simulink model "v01_ssg_only"  (Simulink 7.5)
settings: Solver=ode45  StartTime=0.0  StopTime=128000  RelTol=1e-3
libraries: xbsIndex_r4 x439, xps_library x36, casper_library_misc x18, dspsigops x16, simulink x7
(part 1 of 5)
settings Model: Creator=mwagner  LastModifiedBy=gjones
settings DebuggingCC: StrictBusMsg=Warning

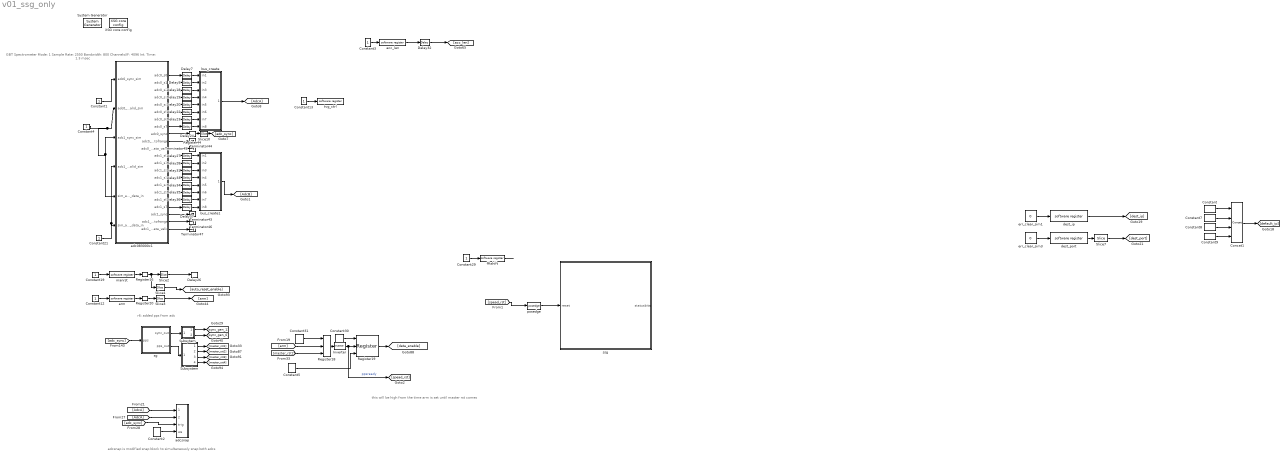
== system v01_ssg_only ==
  note: GBT Spectrometer
      | Mode: 1
      | Sample Rate: 2550
      | Bandwidth: 800
      | Channels/IF: 4096
      | Int. Time: 1.3 msec
  note: r6: added pps from adc
  note: adcsnap is modified snap block to simultaneously snap both adcs
  note: this will be high from the time arm is set until master rst comes
  " System Generator" : xbsIndex_r4/ System Generator  Tag=genX  SystemSampleTime=-1  xilinxfamily=virtex5  part=xc5vsx95t  speed=-1  package=ff1136  synthesis_tool=XST  clock_wrapper=Clock Enables  directory=./v01_ssg_only/sysgen  proj_type=Project Navigator  Synth_file=XST Defaults  Impl_file=ISE Defaults  testbench=off  simulink_period=1  sysclk_period=2.6667  dcm_input_clock_period=100  incr_netlist=off  trim_vbits=Everywhere in SubSystem  dbl_ovrd=According to Block Masks  core_generation=According to Block Masks  run_coregen=off  deprecated_control=off  eval_field=0  block_type=sysgen
      settings: block_version=10.1.3
  Concat1 : xbsIndex_r4/Concat  num_inputs=4  dbl_ovrd=off  block_type=concat
  Constant : xbsIndex_r4/Constant  const=10  gui_display_data_type=Fixed-point  arith_type=Unsigned  n_bits=8  bin_pt=0  preci_type=Single  exp_width=8  frac_width=24  explicit_period=on  period=1  equ=P=C  opselect=C  inp2=PCIN>>17  opr=+  inp1=P  carry=CIN  dbl_ovrd=off  block_type=constant
      settings: block_version=11.4
  Constant1 : Constant  SampleTime=1
  Constant{3,12..13,19,29} (5 alike) : Constant
  Constant{2,5,30..31} (4 alike) : xbsIndex_r4/Constant  const=1  gui_display_data_type=Fixed-point  arith_type=Boolean  n_bits=16  bin_pt=0  preci_type=Single  exp_width=8  frac_width=24  explicit_period=on  period=1  equ=P=C  opselect=C  inp2=PCIN>>17  opr=+  inp1=P  carry=CIN  dbl_ovrd=off  block_type=constant
      settings: block_version=11.4
  Constant21 : Constant  SampleTime=1
  Constant4 : Constant  SampleTime=1
  Constant7 : xbsIndex_r4/Constant  const=0  gui_display_data_type=Fixed-point  arith_type=Unsigned  n_bits=8  bin_pt=0  preci_type=Single  exp_width=8  frac_width=24  explicit_period=on  period=1  equ=P=C  opselect=C  inp2=PCIN>>17  opr=+  inp1=P  carry=CIN  dbl_ovrd=off  block_type=constant
      settings: block_version=11.4
  Constant8 : xbsIndex_r4/Constant  const=0  gui_display_data_type=Fixed-point  arith_type=Unsigned  n_bits=8  bin_pt=0  preci_type=Single  exp_width=8  frac_width=24  explicit_period=on  period=1  equ=P=C  opselect=C  inp2=PCIN>>17  opr=+  inp1=P  carry=CIN  dbl_ovrd=off  block_type=constant
      settings: block_version=11.4
  Constant9 : xbsIndex_r4/Constant  const=145  gui_display_data_type=Fixed-point  arith_type=Unsigned  n_bits=8  bin_pt=0  preci_type=Single  exp_width=8  frac_width=24  explicit_period=on  period=1  equ=P=C  opselect=C  inp2=PCIN>>17  opr=+  inp1=P  carry=CIN  dbl_ovrd=off  block_type=constant
      settings: block_version=11.4
  Delay{7,9,18..20,22..24,27..28,31,33..37} (16 alike) : xbsIndex_r4/Delay  rst=off  infoeditControl=Selection of Reset will increase slice count due to use of real FFs and instead of SRLs  en=off  latency=1  dbl_ovrd=off  reg_retiming=on  block_type=delay
      settings: block_version=11.4
  Delay26 : xbsIndex_r4/Delay  rst=off  infoeditControl=Selection of Reset will increase slice count due to use of real FFs and instead of SRLs  en=off  latency=8  dbl_ovrd=off  reg_retiming=on  block_type=delay
  Delay32 : xbsIndex_r4/Delay  rst=off  infoeditControl=Selection of Reset will increase slice count due to use of real FFs and instead of SRLs  en=off  latency=1  dbl_ovrd=off  reg_retiming=off  block_type=delay
      settings: block_version=11.4
  Inverter : xbsIndex_r4/Inverter  en=off  latency=0  dbl_ovrd=off  block_type=inv
      settings: block_version=11.4
  Register16 : xbsIndex_r4/Register  init=0  rst=off  en=off  dbl_ovrd=off  block_type=register
      settings: block_version=11.4
  Register18 : xbsIndex_r4/Register  init=0  rst=on  en=on  dbl_ovrd=off  block_type=register
      settings: block_version=11.4
  Register19 : xbsIndex_r4/Register  init=0  rst=on  en=on  dbl_ovrd=off  block_type=register
      settings: block_version=11.4
  Register20 : xbsIndex_r4/Register  init=0  rst=off  en=off  dbl_ovrd=off  block_type=register
      settings: block_version=11.4
  Register44 : xbsIndex_r4/Register  init=0  rst=off  en=off  dbl_ovrd=off  block_type=register
      settings: block_version=11.4
  Slice10 : xbsIndex_r4/Slice  nbits=1  boolean_output=on  mode=Lower Bit Location + Width  bit1=0  base1=MSB of Input  bit0=0  base0=LSB of Input  dbl_ovrd=off  block_type=slice
      settings: infoedit="Extracts a given range of bits from each input sample and presents it at the output.  The output type is ordinarily unsigned with binary point at zero, but can be Boolean when the slice is one bit wide.<P><P>Hardware notes: In hardware this block costs nothing."  block_version=10.1.3
  Slice2 : xbsIndex_r4/Slice  nbits=1  boolean_output=on  mode=Lower Bit Location + Width  bit1=0  base1=MSB of Input  bit0=0  base0=LSB of Input  dbl_ovrd=off  block_type=slice
      settings: block_version=10.1.3
  Slice3 : xbsIndex_r4/Slice  nbits=1  boolean_output=on  mode=Lower Bit Location + Width  bit1=0  base1=MSB of Input  bit0=0  base0=LSB of Input  dbl_ovrd=off  block_type=slice
      settings: block_version=10.1.3
  Slice4 : xbsIndex_r4/Slice  nbits=1  boolean_output=on  mode=Lower Bit Location + Width  bit1=0  base1=MSB of Input  bit0=1  base0=LSB of Input  dbl_ovrd=off  block_type=slice
      settings: block_version=10.1.3
  Slice7 : xbsIndex_r4/Slice  nbits=16  boolean_output=off  mode=Lower Bit Location + Width  bit1=0  base1=MSB of Input  bit0=0  base0=LSB of Input  dbl_ovrd=off  block_type=slice
      settings: infoedit="Extracts a given range of bits from each input sample and presents it at the output.  The output type is ordinarily unsigned with binary point at zero, but can be Boolean when the slice is one bit wide.<P><P>Hardware notes: In hardware this block costs nothing."  block_version=10.1.3
  Subsystem : Subsystem
  Subsytem : Subsystem
  Terminator{43..47} (5 alike) : Terminator
  XSG core config : xps_library/XSG core config  Tag=xps:xsg  SystemSampleTime=-1  hw_sys=ROACH:sx95t  ibob_linux=off  clk_src=adc0_clk  iBOB_clk_src=adc0_clk  BEE2_ctrl_clk_src=sys_clk  BEE2_usr_clk_src=sys_clk  ROACH_clk_src=adc0_clk  ROACH2_clk_src=adc0_clk  CORR_clk_src=sys_clk  gpio_clk_io_group=iBOB:sma  gpio_clk_bit_index=0  clk_rate=375  sample_period=1  synthesis_tool=XST  mpc_type=powerpc440_ext
  acc_len : xps_library/software register  Tag=xps:sw_reg  SystemSampleTime=-1  io_dir=From Processor  arith_type=Unsigned  bitwidth=32  bin_pt=0  sample_period=1  gw_name=v01_ssg_only_acc_len_user_data_out
      link override convert: arith_type=Unsigned  n_bits=32  bin_pt=0
      link override r_spec_2048_r102_cnt_rst_user_data_out: arith_type=Unsigned  n_bits=32  bin_pt=0  period=1
      link override r_spec_2048_r102_nosim_cnt_rst_user_data_out: arith_type=Unsigned  n_bits=32  bin_pt=0  period=1
      link override r_spec_2048_r103_cnt_rst_user_data_out: arith_type=Unsigned  n_bits=32  bin_pt=0  period=1
      link override roach_spec_no10gbe_sync_cnt_rst_user_data_out: arith_type=Unsigned  n_bits=32  bin_pt=0  period=1
      link override roach_spec_rst_cnt_user_data_out: arith_type=Unsigned  n_bits=32  bin_pt=0  period=1
      link override roach_spec_rst_sync_cnt_user_data_out: arith_type=Unsigned  n_bits=32  bin_pt=0  period=1
  adc083000x1 : Subsystem  Tag=xps:adc083000x2  AncestorBlock=xps_library/adc083000x2  mask(adc_083000x2){use_adc0=on, use_adc1=on, demux_adc=off, clock_sync=off, verbose=off, using_ctrl=on, adc_clk_rate=1500, sample_period=1, bit_width=8}
      mask prompts: use_adc0 "Use ZD0K0?"; use_adc1 "Use ZDOK1?"; demux_adc "Demux ADCs by 2?"; clock_sync "Interleave 2 ADC boards?"; verbose "Verbose Block Creation?"; using_ctrl "Add ports for control registers?"; adc_clk_rate "ADC clock rate (MHz)"; sample_period "Sample Period"; bit_width "Output Bit Width"
      mask help:
      | The ADC block converts analog inputs to digital outputs.
      | Every clock cycle, the inputs are sampled and digitized to
      | 8 bit binary point numbers in the range of [-1, 1).
      |
      | Online block-specific documentation: http://casper.berkeley.edu/wiki/Adc083000
      mask init:
      | adc083000_mask;
      mask Help: eval('xlWeb([getenv(''MLIB_ROOT''), ''\doc\html\sys_adc\sys_adc.html''])')
  adcsnap : Subsystem  mask(snap64){nsamples=11}
      mask prompts: nsamples "No. of samples(2^?)"
      mask help:
      | The <i>snap</i> block provides a packaged solution to capturing data from
      | the FPGA fabric and making it accessible from the CPU.  The block comes in
      | 2 flavors: <i>snap</i> (which captures to a 32 bit wide Shared BRAM), and
      | <i>snap64</i> (which captures to 2x32 bit wide Shared BRAMs to effect a
      | 64 bit capture).
      mask Help: eval('xlWeb(''http://casper.berkeley.edu/wiki/Snap'')')
  arm : xps_library/software register  Tag=xps:sw_reg  SystemSampleTime=-1  io_dir=From Processor  arith_type=Unsigned  bitwidth=32  bin_pt=0  sample_period=1  gw_name=v01_ssg_only_arm_user_data_out
      link override convert: arith_type=Unsigned  n_bits=32  bin_pt=0
      link override r_spec_2048_r102_cnt_rst_user_data_out: arith_type=Unsigned  n_bits=32  bin_pt=0  period=1
      link override r_spec_2048_r102_nosim_cnt_rst_user_data_out: arith_type=Unsigned  n_bits=32  bin_pt=0  period=1
      link override r_spec_2048_r103_cnt_rst_user_data_out: arith_type=Unsigned  n_bits=32  bin_pt=0  period=1
      link override roach_spec_no10gbe_sync_cnt_rst_user_data_out: arith_type=Unsigned  n_bits=32  bin_pt=0  period=1
      link override roach_spec_rst_cnt_user_data_out: arith_type=Unsigned  n_bits=32  bin_pt=0  period=1
      link override roach_spec_rst_sync_cnt_user_data_out: arith_type=Unsigned  n_bits=32  bin_pt=0  period=1
  bus_create : Subsystem  AncestorBlock=casper_library_flow_control/bus_create  mask(bus_create){inputNum=8}
      mask prompts: inputNum "Number of inputs:"
      mask init:
      | bus_create_init(gcb,...
      |     'inputNum', inputNum);
  bus_create1 : Subsystem  AncestorBlock=casper_library_flow_control/bus_create  mask(bus_create){inputNum=8}
      mask prompts: inputNum "Number of inputs:"
      mask init:
      | bus_create_init(gcb,...
      |     'inputNum', inputNum);
  dest_ip : xps_library/software register  Tag=xps:sw_reg  SystemSampleTime=-1  io_dir=From Processor  arith_type=Unsigned  bitwidth=32  bin_pt=0  sample_period=1  gw_name=v01_ssg_only_dest_ip_user_data_out
      link override r_10gbe_demo_dest_ip_user_data_out: arith_type=Unsigned  n_bits=32  bin_pt=0  period=1
      link override r_10gbe_test_dest_ip_user_data_out: arith_type=Unsigned  n_bits=32  bin_pt=0  period=1
      link override r_xaui_test_cnt_rst_user_data_out: arith_type=Unsigned  n_bits=32  bin_pt=0  period=1
  dest_port : xps_library/software register  Tag=xps:sw_reg  SystemSampleTime=-1  io_dir=From Processor  arith_type=Unsigned  bitwidth=32  bin_pt=0  sample_period=1  gw_name=v01_ssg_only_dest_port_user_data_out
      link override r_10gbe_demo_dest_port_user_data_out: arith_type=Unsigned  n_bits=32  bin_pt=0  period=1
      link override r_10gbe_test_dest_port_user_data_out: arith_type=Unsigned  n_bits=32  bin_pt=0  period=1
      link override r_xaui_test_cnt_rst_user_data_out: arith_type=Unsigned  n_bits=32  bin_pt=0  period=1
  err_clear_sim1 : Constant  Value=0
  err_clear_sim3 : Constant  Value=0
  fftshift : xps_library/software register  Tag=xps:sw_reg  SystemSampleTime=-1  io_dir=From Processor  arith_type=Unsigned  bitwidth=32  bin_pt=0  sample_period=1  gw_name=v01_ssg_only_fftshift_user_data_out
  manrst : xps_library/software register  Tag=xps:sw_reg  SystemSampleTime=-1  io_dir=From Processor  arith_type=Unsigned  bitwidth=32  bin_pt=0  sample_period=1  gw_name=v01_ssg_only_manrst_user_data_out
      link override convert: arith_type=Unsigned  n_bits=32  bin_pt=0
      link override r_spec_2048_r102_cnt_rst_user_data_out: arith_type=Unsigned  n_bits=32  bin_pt=0  period=1
      link override r_spec_2048_r102_nosim_cnt_rst_user_data_out: arith_type=Unsigned  n_bits=32  bin_pt=0  period=1
      link override r_spec_2048_r103_cnt_rst_user_data_out: arith_type=Unsigned  n_bits=32  bin_pt=0  period=1
      link override roach_spec_no10gbe_sync_cnt_rst_user_data_out: arith_type=Unsigned  n_bits=32  bin_pt=0  period=1
      link override roach_spec_rst_cnt_user_data_out: arith_type=Unsigned  n_bits=32  bin_pt=0  period=1
      link override roach_spec_rst_sync_cnt_user_data_out: arith_type=Unsigned  n_bits=32  bin_pt=0  period=1
  posedge : casper_library_misc/posedge  Tag=Rising Edge Detector  SystemSampleTime=-1
  sg : Subsystem
  ssg : Subsystem
  tvg_ctrl : xps_library/software register  Tag=xps:sw_reg  SystemSampleTime=-1  io_dir=From Processor  arith_type=Unsigned  bitwidth=32  bin_pt=0  sample_period=1  gw_name=v01_ssg_only_tvg_ctrl_user_data_out
      link override convert: arith_type=Unsigned  n_bits=32  bin_pt=0
      link override r_spec_2048_r102_cnt_rst_user_data_out: arith_type=Unsigned  n_bits=32  bin_pt=0  period=1
      link override r_spec_2048_r102_nosim_cnt_rst_user_data_out: arith_type=Unsigned  n_bits=32  bin_pt=0  period=1
      link override r_spec_2048_r103_cnt_rst_user_data_out: arith_type=Unsigned  n_bits=32  bin_pt=0  period=1
      link override roach_spec_no10gbe_sync_cnt_rst_user_data_out: arith_type=Unsigned  n_bits=32  bin_pt=0  period=1
      link override roach_spec_rst_cnt_user_data_out: arith_type=Unsigned  n_bits=32  bin_pt=0  period=1
      link override roach_spec_rst_sync_cnt_user_data_out: arith_type=Unsigned  n_bits=32  bin_pt=0  period=1
  wires:
  manrst/1 -> Register16/1
  Constant19/1 -> manrst/1
  Register16/1 -> Slice2/1, Slice4/1
  Slice2/1 -> Delay26/1
  Constant4/1 -> adc083000x1/2(adc0_data_valid_sim), adc083000x1/3(adc1_sync_sim), adc083000x1/5(sim_adc0_data_in)
  Constant1/1 -> adc083000x1/1(adc0_sync_sim)
  Slice10/1 -> [adc_sync]
  Register44/1 -> Slice10/1
  Constant21/1 -> adc083000x1/4(adc1_data_valid_sim), adc083000x1/6(sim_adc1_data_in)
  Concat1/1 -> [default_ip]
  acc_len/1 -> Delay32/1
  Constant3/1 -> acc_len/1
  Delay32/1 -> [acc_len]
  err_clear_sim1/1 -> dest_ip/1
  dest_ip/1 -> [dest_ip]
  dest_port/1 -> Slice7/1
  err_clear_sim3/1 -> dest_port/1
  Slice7/1 -> [dest_port]
  Constant/1 -> Concat1/1
  Constant7/1 -> Concat1/2
  Constant8/1 -> Concat1/3
  Constant9/1 -> Concat1/4
  Constant30/1 -> Register19/1
  Register18/1 -> Inverter/1
  Inverter/1 -> Register19/2, [spead_rst]  "ppsready"
  Constant31/1 -> Register18/1
  arm/1 -> Register20/1
  Constant12/1 -> arm/1
  Register20/1 -> Slice3/1
  Slice3/1 -> [arm]
  [arm] -> Register18/2
  [master_rst2] -> Register18/3
  Constant5/1 -> Register19/3
  Register19/1 -> [data_enable]
  [adc_sync] -> sg/1(pps)
  Slice4/1 -> [auto_reset_enable]
  sg/1(sync_out) -> Subsytem/1(In1)
  Subsytem/1(Out1) -> [sync_gen_1]
  Subsytem/2(Out2) -> [sync_gen_0]
  Delay7/1 -> bus_create/1(in1)
  Delay9/1 -> bus_create/2(in2)
  Delay18/1 -> bus_create/3(in3)
  Delay19/1 -> bus_create/4(in4)
  Delay20/1 -> bus_create/5(in5)
  Delay22/1 -> bus_create/6(in6)
  Delay23/1 -> bus_create/7(in7)
  Delay24/1 -> bus_create/8(in8)
  Delay27/1 -> bus_create1/1(in1)
  Delay28/1 -> bus_create1/2(in2)
  Delay31/1 -> bus_create1/3(in3)
  Delay33/1 -> bus_create1/4(in4)
  Delay34/1 -> bus_create1/5(in5)
  Delay35/1 -> bus_create1/6(in6)
  Delay36/1 -> bus_create1/7(in7)
  Delay37/1 -> bus_create1/8(in8)
  sg/2(pps_out) -> Subsystem/1(In2)
  Subsystem/1(Out1) -> [master_rst1]
  Subsystem/2(Out2) -> [master_rst2]
  Subsystem/3(Out3) -> [master_rst3]
  Subsystem/4(Out4) -> [master_rst4]
  adc083000x1/1(adc0_s0) -> Delay7/1
  adc083000x1/2(adc0_s1) -> Delay9/1
  adc083000x1/3(adc0_s2) -> Delay18/1
  adc083000x1/4(adc0_s3) -> Delay19/1
  adc083000x1/5(adc0_s4) -> Delay20/1
  adc083000x1/6(adc0_s5) -> Delay22/1
  adc083000x1/7(adc0_s6) -> Delay23/1
  adc083000x1/8(adc0_s7) -> Delay24/1
  adc083000x1/9(adc0_sync) -> Register44/1
  adc083000x1/10(adc0_outofrange) -> Terminator44/1
  adc083000x1/11(adc0_data_valid) -> Terminator45/1
  adc083000x1/12(adc1_s0) -> Delay27/1
  adc083000x1/13(adc1_s1) -> Delay28/1
  adc083000x1/14(adc1_s2) -> Delay31/1
  adc083000x1/15(adc1_s3) -> Delay33/1
  adc083000x1/16(adc1_s4) -> Delay34/1
  adc083000x1/17(adc1_s5) -> Delay35/1
  adc083000x1/18(adc1_s6) -> Delay36/1
  adc083000x1/19(adc1_s7) -> Delay37/1
  adc083000x1/20(adc1_sync) -> Terminator43/1
  adc083000x1/21(adc1_outofrange) -> Terminator46/1
  adc083000x1/22(adc1_data_valid) -> Terminator47/1
  Constant13/1 -> tvg_ctrl/1
  bus_create/1(bus_out) -> [AdcA]
  bus_create1/1(bus_out) -> [AdcB]
  Constant29/1 -> fftshift/1
  fftshift/1 -> ?
  [AdcA] -> adcsnap/1(adcA)
  [AdcA] -> adcsnap/2(adcB)
  [adc_sync] -> adcsnap/3(trig)
  Constant2/1 -> adcsnap/4(we)
  ? -> ?
  ? -> ?
  ? -> ?
  [spead_rst] -> posedge/1
  posedge/1 -> ssg/1(reset)

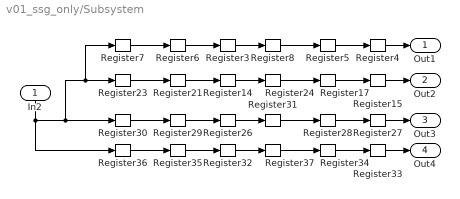
== system v01_ssg_only/Subsystem ==
  In2 : Inport
  Register{3..8,14..15,17,21,23..24,26..37} (24 alike) : xbsIndex_r4/Register  init=0  rst=off  en=off  dbl_ovrd=off  block_type=register
      settings: block_version=11.4
  Out1 : Outport
  Out2 : Outport  Port=2
  Out3 : Outport  Port=3
  Out4 : Outport  Port=4
  wires:
  Register7/1 -> Register6/1
  Register6/1 -> Register3/1
  Register8/1 -> Register5/1
  Register5/1 -> Register4/1
  Register3/1 -> Register8/1
  Register23/1 -> Register21/1
  Register21/1 -> Register14/1
  Register24/1 -> Register17/1
  Register17/1 -> Register15/1
  Register14/1 -> Register24/1
  Register30/1 -> Register29/1
  Register29/1 -> Register26/1
  Register31/1 -> Register28/1
  Register28/1 -> Register27/1
  Register26/1 -> Register31/1
  Register36/1 -> Register35/1
  Register35/1 -> Register32/1
  Register37/1 -> Register34/1
  Register34/1 -> Register33/1
  Register32/1 -> Register37/1
  In2/1 -> Register36/1, Register30/1, Register23/1, Register7/1
  Register4/1 -> Out1/1
  Register15/1 -> Out2/1
  Register27/1 -> Out3/1
  Register33/1 -> Out4/1

== system v01_ssg_only/Subsytem ==
  In1 : Inport
  Register{3..8,14..15,17} (9 alike) : xbsIndex_r4/Register  init=0  rst=off  en=off  dbl_ovrd=off  block_type=register
      settings: block_version=11.4
  Out1 : Outport
  Out2 : Outport  Port=2
  wires:
  Register3/1 -> Register4/1, Register5/1
  Register7/1 -> Register6/1
  Register6/1 -> Register3/1
  Register5/1 -> Register14/1
  Register4/1 -> Register8/1
  Register8/1 -> Register17/1
  Register14/1 -> Register15/1
  Register17/1 -> Out1/1
  In1/1 -> Register7/1
  Register15/1 -> Out2/1

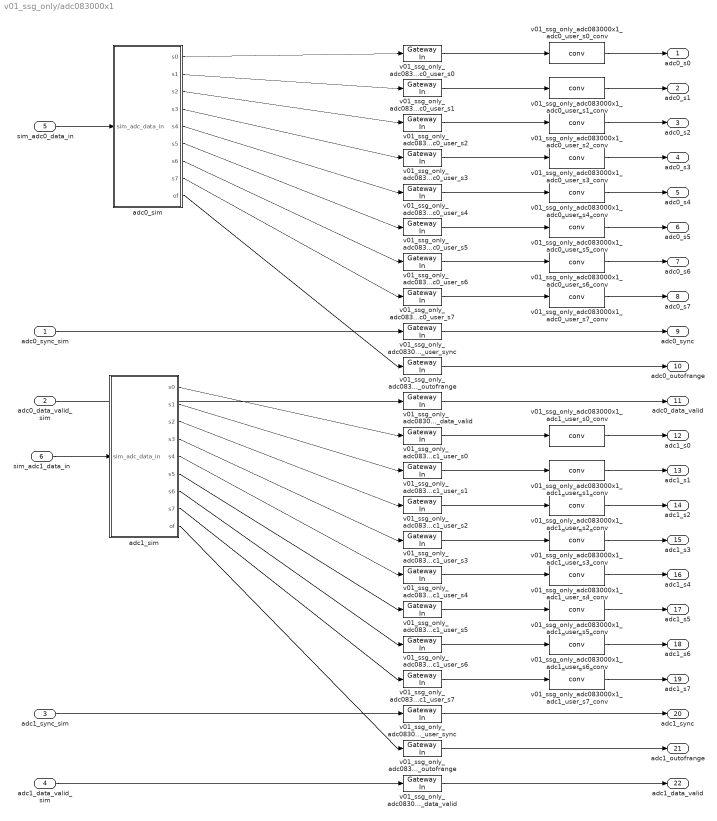
== system v01_ssg_only/adc083000x1 ==
  adc0_sync_sim : Inport
  adc0_data_valid_sim : Inport  Port=2
  adc1_sync_sim : Inport  Port=3
  adc1_data_valid_sim : Inport  Port=4
  sim_adc0_data_in : Inport  Port=5
  sim_adc1_data_in : Inport  Port=6
  adc0_sim : Subsystem  AncestorBlock=xps_library/ADCs/adc_sim  mask(adc_sim){nStreams=8, bit_width=8}
      mask prompts: nStreams "Number of Output Streams"; bit_width "Sample Bit Width"
      mask help:
      | This block simulates the behavior of a demuxed ADC, which takes
      | as input a waveform and returns digital samples in parallel at
      | a slower rate.
      |
      | This block is used to simulate the behavior
      mask init:
      | adc_sim_init(gcb, ...
      |     'nStreams', nStreams, ...
      |     'bit_width', bit_width);
  adc1_sim : Subsystem  AncestorBlock=xps_library/ADCs/adc_sim  mask(adc_sim){nStreams=8, bit_width=8}
      mask prompts: nStreams "Number of Output Streams"; bit_width "Sample Bit Width"
      mask help:
      | This block simulates the behavior of a demuxed ADC, which takes
      | as input a waveform and returns digital samples in parallel at
      | a slower rate.
      |
      | This block is used to simulate the behavior
      mask init:
      | adc_sim_init(gcb, ...
      |     'nStreams', nStreams, ...
      |     'bit_width', bit_width);
  v01_ssg_only_adc083000x1_adc0_user_data_valid : xbsIndex_r4/Gateway In  gui_display_data_type=Fixed-point  arith_type=Unsigned  n_bits=1  bin_pt=0  preci_type=Single  exp_width=8  frac_width=24  quantization="Round  (unbiased: +/- Inf)"  overflow=Saturate  period=1  dbl_ovrd=off  timing_constraint=None  locs_specified=off  LOCs={}  hdl_port=on  block_type=gatewayin
      settings: infoedit="Gateway in block.  Converts inputs of type Simulink integer, double and fixed point to  Xilinx fixed point or floating-point data type.<br><br>Hardware notes:  In hardware these blocks become top level input ports."
  v01_ssg_only_adc083000x1_adc0_user_outofrange : xbsIndex_r4/Gateway In  gui_display_data_type=Fixed-point  arith_type=Unsigned  n_bits=4  bin_pt=0  preci_type=Single  exp_width=8  frac_width=24  quantization="Round  (unbiased: +/- Inf)"  overflow=Saturate  period=1  dbl_ovrd=off  timing_constraint=None  locs_specified=off  LOCs={}  hdl_port=on  block_type=gatewayin
      settings: infoedit="Gateway in block.  Converts inputs of type Simulink integer, double and fixed point to  Xilinx fixed point or floating-point data type.<br><br>Hardware notes:  In hardware these blocks become top level input ports."
  v01_ssg_only_adc083000x1_adc0_user_s{0..7} (8 alike) : xbsIndex_r4/Gateway In  gui_display_data_type=Fixed-point  arith_type=Unsigned  n_bits=8  bin_pt=0  preci_type=Single  exp_width=8  frac_width=24  quantization="Round  (unbiased: +/- Inf)"  overflow=Saturate  period=1  dbl_ovrd=off  timing_constraint=None  locs_specified=off  LOCs={}  hdl_port=on  block_type=gatewayin
      settings: infoedit="Gateway in block.  Converts inputs of type Simulink integer, double and fixed point to  Xilinx fixed point or floating-point data type.<br><br>Hardware notes:  In hardware these blocks become top level input ports."
  v01_ssg_only_adc083000x1_adc0_user_s0_conv : xps_library/ADCs/conv  SystemSampleTime=-1  bit_width=8
  v01_ssg_only_adc083000x1_adc0_user_s1_conv : xps_library/ADCs/conv  SystemSampleTime=-1  bit_width=8
  v01_ssg_only_adc083000x1_adc0_user_s2_conv : xps_library/ADCs/conv  SystemSampleTime=-1  bit_width=8
  v01_ssg_only_adc083000x1_adc0_user_s3_conv : xps_library/ADCs/conv  SystemSampleTime=-1  bit_width=8
  v01_ssg_only_adc083000x1_adc0_user_s4_conv : xps_library/ADCs/conv  SystemSampleTime=-1  bit_width=8
  v01_ssg_only_adc083000x1_adc0_user_s5_conv : xps_library/ADCs/conv  SystemSampleTime=-1  bit_width=8
  v01_ssg_only_adc083000x1_adc0_user_s6_conv : xps_library/ADCs/conv  SystemSampleTime=-1  bit_width=8
  v01_ssg_only_adc083000x1_adc0_user_s7_conv : xps_library/ADCs/conv  SystemSampleTime=-1  bit_width=8
  v01_ssg_only_adc083000x1_adc0_user_sync : xbsIndex_r4/Gateway In  gui_display_data_type=Fixed-point  arith_type=Unsigned  n_bits=4  bin_pt=0  preci_type=Single  exp_width=8  frac_width=24  quantization="Round  (unbiased: +/- Inf)"  overflow=Saturate  period=1  dbl_ovrd=off  timing_constraint=None  locs_specified=off  LOCs={}  hdl_port=on  block_type=gatewayin
      settings: infoedit="Gateway in block.  Converts inputs of type Simulink integer, double and fixed point to  Xilinx fixed point or floating-point data type.<br><br>Hardware notes:  In hardware these blocks become top level input ports."
  v01_ssg_only_adc083000x1_adc1_user_data_valid : xbsIndex_r4/Gateway In  gui_display_data_type=Fixed-point  arith_type=Unsigned  n_bits=1  bin_pt=0  preci_type=Single  exp_width=8  frac_width=24  quantization="Round  (unbiased: +/- Inf)"  overflow=Saturate  period=1  dbl_ovrd=off  timing_constraint=None  locs_specified=off  LOCs={}  hdl_port=on  block_type=gatewayin
      settings: infoedit="Gateway in block.  Converts inputs of type Simulink integer, double and fixed point to  Xilinx fixed point or floating-point data type.<br><br>Hardware notes:  In hardware these blocks become top level input ports."
  v01_ssg_only_adc083000x1_adc1_user_outofrange : xbsIndex_r4/Gateway In  gui_display_data_type=Fixed-point  arith_type=Unsigned  n_bits=4  bin_pt=0  preci_type=Single  exp_width=8  frac_width=24  quantization="Round  (unbiased: +/- Inf)"  overflow=Saturate  period=1  dbl_ovrd=off  timing_constraint=None  locs_specified=off  LOCs={}  hdl_port=on  block_type=gatewayin
      settings: infoedit="Gateway in block.  Converts inputs of type Simulink integer, double and fixed point to  Xilinx fixed point or floating-point data type.<br><br>Hardware notes:  In hardware these blocks become top level input ports."
  v01_ssg_only_adc083000x1_adc1_user_s{0..7} (8 alike) : xbsIndex_r4/Gateway In  gui_display_data_type=Fixed-point  arith_type=Unsigned  n_bits=8  bin_pt=0  preci_type=Single  exp_width=8  frac_width=24  quantization="Round  (unbiased: +/- Inf)"  overflow=Saturate  period=1  dbl_ovrd=off  timing_constraint=None  locs_specified=off  LOCs={}  hdl_port=on  block_type=gatewayin
      settings: infoedit="Gateway in block.  Converts inputs of type Simulink integer, double and fixed point to  Xilinx fixed point or floating-point data type.<br><br>Hardware notes:  In hardware these blocks become top level input ports."
  v01_ssg_only_adc083000x1_adc1_user_s0_conv : xps_library/ADCs/conv  SystemSampleTime=-1  bit_width=8
  v01_ssg_only_adc083000x1_adc1_user_s1_conv : xps_library/ADCs/conv  SystemSampleTime=-1  bit_width=8
  v01_ssg_only_adc083000x1_adc1_user_s2_conv : xps_library/ADCs/conv  SystemSampleTime=-1  bit_width=8
  v01_ssg_only_adc083000x1_adc1_user_s3_conv : xps_library/ADCs/conv  SystemSampleTime=-1  bit_width=8
  v01_ssg_only_adc083000x1_adc1_user_s4_conv : xps_library/ADCs/conv  SystemSampleTime=-1  bit_width=8
  v01_ssg_only_adc083000x1_adc1_user_s5_conv : xps_library/ADCs/conv  SystemSampleTime=-1  bit_width=8
  v01_ssg_only_adc083000x1_adc1_user_s6_conv : xps_library/ADCs/conv  SystemSampleTime=-1  bit_width=8
  v01_ssg_only_adc083000x1_adc1_user_s7_conv : xps_library/ADCs/conv  SystemSampleTime=-1  bit_width=8
  v01_ssg_only_adc083000x1_adc1_user_sync : xbsIndex_r4/Gateway In  gui_display_data_type=Fixed-point  arith_type=Unsigned  n_bits=4  bin_pt=0  preci_type=Single  exp_width=8  frac_width=24  quantization="Round  (unbiased: +/- Inf)"  overflow=Saturate  period=1  dbl_ovrd=off  timing_constraint=None  locs_specified=off  LOCs={}  hdl_port=on  block_type=gatewayin
      settings: infoedit="Gateway in block.  Converts inputs of type Simulink integer, double and fixed point to  Xilinx fixed point or floating-point data type.<br><br>Hardware notes:  In hardware these blocks become top level input ports."
  adc0_s0 : Outport
  adc0_s1 : Outport  Port=2
  adc0_s2 : Outport  Port=3
  adc0_s3 : Outport  Port=4
  adc0_s4 : Outport  Port=5
  adc0_s5 : Outport  Port=6
  adc0_s6 : Outport  Port=7
  adc0_s7 : Outport  Port=8
  adc0_sync : Outport  Port=9
  adc0_outofrange : Outport  Port=10
  adc0_data_valid : Outport  Port=11
  adc1_s0 : Outport  Port=12
  adc1_s1 : Outport  Port=13
  adc1_s2 : Outport  Port=14
  adc1_s3 : Outport  Port=15
  adc1_s4 : Outport  Port=16
  adc1_s5 : Outport  Port=17
  adc1_s6 : Outport  Port=18
  adc1_s7 : Outport  Port=19
  adc1_sync : Outport  Port=20
  adc1_outofrange : Outport  Port=21
  adc1_data_valid : Outport  Port=22
  wires:
  sim_adc0_data_in/1 -> adc0_sim/1(sim_adc_data_in)
  sim_adc1_data_in/1 -> adc1_sim/1(sim_adc_data_in)
  adc0_sim/1(s0) -> v01_ssg_only_adc083000x1_adc0_user_s0/1
  v01_ssg_only_adc083000x1_adc0_user_s0/1 -> v01_ssg_only_adc083000x1_adc0_user_s0_conv/1
  v01_ssg_only_adc083000x1_adc0_user_s0_conv/1 -> adc0_s0/1
  adc0_sim/2(s1) -> v01_ssg_only_adc083000x1_adc0_user_s1/1
  v01_ssg_only_adc083000x1_adc0_user_s1/1 -> v01_ssg_only_adc083000x1_adc0_user_s1_conv/1
  v01_ssg_only_adc083000x1_adc0_user_s1_conv/1 -> adc0_s1/1
  adc0_sim/3(s2) -> v01_ssg_only_adc083000x1_adc0_user_s2/1
  v01_ssg_only_adc083000x1_adc0_user_s2/1 -> v01_ssg_only_adc083000x1_adc0_user_s2_conv/1
  v01_ssg_only_adc083000x1_adc0_user_s2_conv/1 -> adc0_s2/1
  adc0_sim/4(s3) -> v01_ssg_only_adc083000x1_adc0_user_s3/1
  v01_ssg_only_adc083000x1_adc0_user_s3/1 -> v01_ssg_only_adc083000x1_adc0_user_s3_conv/1
  v01_ssg_only_adc083000x1_adc0_user_s3_conv/1 -> adc0_s3/1
  adc0_sim/5(s4) -> v01_ssg_only_adc083000x1_adc0_user_s4/1
  v01_ssg_only_adc083000x1_adc0_user_s4/1 -> v01_ssg_only_adc083000x1_adc0_user_s4_conv/1
  v01_ssg_only_adc083000x1_adc0_user_s4_conv/1 -> adc0_s4/1
  adc0_sim/6(s5) -> v01_ssg_only_adc083000x1_adc0_user_s5/1
  v01_ssg_only_adc083000x1_adc0_user_s5/1 -> v01_ssg_only_adc083000x1_adc0_user_s5_conv/1
  v01_ssg_only_adc083000x1_adc0_user_s5_conv/1 -> adc0_s5/1
  adc0_sim/7(s6) -> v01_ssg_only_adc083000x1_adc0_user_s6/1
  v01_ssg_only_adc083000x1_adc0_user_s6/1 -> v01_ssg_only_adc083000x1_adc0_user_s6_conv/1
  v01_ssg_only_adc083000x1_adc0_user_s6_conv/1 -> adc0_s6/1
  adc0_sim/8(s7) -> v01_ssg_only_adc083000x1_adc0_user_s7/1
  v01_ssg_only_adc083000x1_adc0_user_s7/1 -> v01_ssg_only_adc083000x1_adc0_user_s7_conv/1
  v01_ssg_only_adc083000x1_adc0_user_s7_conv/1 -> adc0_s7/1
  adc0_sync_sim/1 -> v01_ssg_only_adc083000x1_adc0_user_sync/1
  v01_ssg_only_adc083000x1_adc0_user_sync/1 -> adc0_sync/1
  adc0_sim/9(of) -> v01_ssg_only_adc083000x1_adc0_user_outofrange/1
  v01_ssg_only_adc083000x1_adc0_user_outofrange/1 -> adc0_outofrange/1
  adc0_data_valid_sim/1 -> v01_ssg_only_adc083000x1_adc0_user_data_valid/1
  v01_ssg_only_adc083000x1_adc0_user_data_valid/1 -> adc0_data_valid/1
  adc1_sim/1(s0) -> v01_ssg_only_adc083000x1_adc1_user_s0/1
  v01_ssg_only_adc083000x1_adc1_user_s0/1 -> v01_ssg_only_adc083000x1_adc1_user_s0_conv/1
  v01_ssg_only_adc083000x1_adc1_user_s0_conv/1 -> adc1_s0/1
  adc1_sim/2(s1) -> v01_ssg_only_adc083000x1_adc1_user_s1/1
  v01_ssg_only_adc083000x1_adc1_user_s1/1 -> v01_ssg_only_adc083000x1_adc1_user_s1_conv/1
  v01_ssg_only_adc083000x1_adc1_user_s1_conv/1 -> adc1_s1/1
  adc1_sim/3(s2) -> v01_ssg_only_adc083000x1_adc1_user_s2/1
  v01_ssg_only_adc083000x1_adc1_user_s2/1 -> v01_ssg_only_adc083000x1_adc1_user_s2_conv/1
  v01_ssg_only_adc083000x1_adc1_user_s2_conv/1 -> adc1_s2/1
  adc1_sim/4(s3) -> v01_ssg_only_adc083000x1_adc1_user_s3/1
  v01_ssg_only_adc083000x1_adc1_user_s3/1 -> v01_ssg_only_adc083000x1_adc1_user_s3_conv/1
  v01_ssg_only_adc083000x1_adc1_user_s3_conv/1 -> adc1_s3/1
  adc1_sim/5(s4) -> v01_ssg_only_adc083000x1_adc1_user_s4/1
  v01_ssg_only_adc083000x1_adc1_user_s4/1 -> v01_ssg_only_adc083000x1_adc1_user_s4_conv/1
  v01_ssg_only_adc083000x1_adc1_user_s4_conv/1 -> adc1_s4/1
  adc1_sim/6(s5) -> v01_ssg_only_adc083000x1_adc1_user_s5/1
  v01_ssg_only_adc083000x1_adc1_user_s5/1 -> v01_ssg_only_adc083000x1_adc1_user_s5_conv/1
  v01_ssg_only_adc083000x1_adc1_user_s5_conv/1 -> adc1_s5/1
  adc1_sim/7(s6) -> v01_ssg_only_adc083000x1_adc1_user_s6/1
  v01_ssg_only_adc083000x1_adc1_user_s6/1 -> v01_ssg_only_adc083000x1_adc1_user_s6_conv/1
  v01_ssg_only_adc083000x1_adc1_user_s6_conv/1 -> adc1_s6/1
  adc1_sim/8(s7) -> v01_ssg_only_adc083000x1_adc1_user_s7/1
  v01_ssg_only_adc083000x1_adc1_user_s7/1 -> v01_ssg_only_adc083000x1_adc1_user_s7_conv/1
  v01_ssg_only_adc083000x1_adc1_user_s7_conv/1 -> adc1_s7/1
  adc1_sync_sim/1 -> v01_ssg_only_adc083000x1_adc1_user_sync/1
  v01_ssg_only_adc083000x1_adc1_user_sync/1 -> adc1_sync/1
  adc1_sim/9(of) -> v01_ssg_only_adc083000x1_adc1_user_outofrange/1
  v01_ssg_only_adc083000x1_adc1_user_outofrange/1 -> adc1_outofrange/1
  adc1_data_valid_sim/1 -> v01_ssg_only_adc083000x1_adc1_user_data_valid/1
  v01_ssg_only_adc083000x1_adc1_user_data_valid/1 -> adc1_data_valid/1

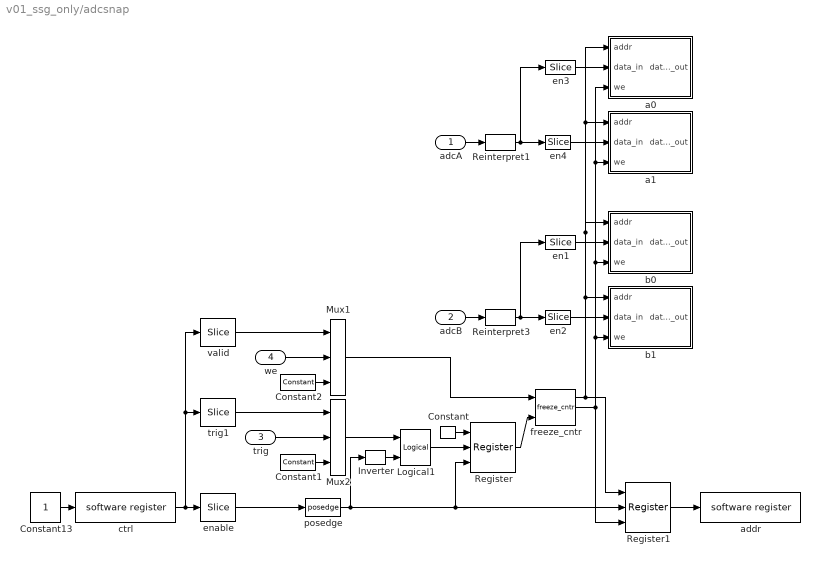
== system v01_ssg_only/adcsnap ==
  adcA : Inport
  adcB : Inport  Port=2
  trig : Inport  Port=3
  we : Inport  Port=4
  Constant : xbsIndex_r4/Constant  const=1  gui_display_data_type=Fixed-point  arith_type=Boolean  n_bits=1  bin_pt=0  preci_type=Single  exp_width=8  frac_width=24  explicit_period=on  period=1  equ=P=C  opselect=C  inp2=PCIN>>17  opr=+  inp1=P  carry=CIN  dbl_ovrd=off  block_type=constant
      settings: block_version=10.1.1
  Constant1 : xbsIndex_r4/Constant  const=1  gui_display_data_type=Fixed-point  arith_type=Boolean  n_bits=1  bin_pt=0  preci_type=Single  exp_width=8  frac_width=24  explicit_period=on  period=1  equ=P=C  opselect=C  inp2=PCIN>>17  opr=+  inp1=P  carry=CIN  dbl_ovrd=off  block_type=constant
      settings: block_version=10.1.1
  Constant13 : Constant
  Constant2 : xbsIndex_r4/Constant  const=1  gui_display_data_type=Fixed-point  arith_type=Boolean  n_bits=1  bin_pt=0  preci_type=Single  exp_width=8  frac_width=24  explicit_period=on  period=1  equ=P=C  opselect=C  inp2=PCIN>>17  opr=+  inp1=P  carry=CIN  dbl_ovrd=off  block_type=constant
      settings: block_version=10.1.1
  Inverter : xbsIndex_r4/Inverter  en=off  latency=0  dbl_ovrd=off  block_type=inv
      settings: xl_area=[0, 0, 0, 0, 0, 0, 0]  block_version=10.1.1
  Logical1 : xbsIndex_r4/Logical  logical_function=AND  inputs=2  en=off  latency=0  precision=Full  arith_type=Unsigned  n_bits=8  bin_pt=2  align_bp=on  dbl_ovrd=off  block_type=logical
      settings: xl_area=[0, 0, 0, 0, 0, 0, 0]  block_version=10.1.1
  Mux1 : xbsIndex_r4/Mux  inputs=2  en=off  latency=0  precision=Full  arith_type="Signed  (2's comp)"  n_bits=8  bin_pt=2  quantization=Truncate  overflow=Wrap  dbl_ovrd=off  block_type=mux
      settings: xl_area=[0, 0, 0, 0, 0, 0, 0]  block_version=10.1.1
  Mux2 : xbsIndex_r4/Mux  inputs=2  en=off  latency=0  precision=Full  arith_type="Signed  (2's comp)"  n_bits=8  bin_pt=2  quantization=Truncate  overflow=Wrap  dbl_ovrd=off  block_type=mux
      settings: xl_area=[0, 0, 0, 0, 0, 0, 0]  block_version=10.1.1
  Register : xbsIndex_r4/Register  init=0  rst=on  en=on  dbl_ovrd=off  block_type=register
      settings: xl_area=[0, 0, 0, 0, 0, 0, 0]  block_version=10.1.1
  Register1 : xbsIndex_r4/Register  init=0  rst=on  en=on  dbl_ovrd=off  block_type=register
      settings: xl_area=[0, 0, 0, 0, 0, 0, 0]  block_version=10.1.1
  Reinterpret1 : xbsIndex_r4/Reinterpret  force_arith_type=on  arith_type=Unsigned  force_bin_pt=on  bin_pt=0  block_type=reinterpret
      settings: infoedit="Changes signal type without altering the binary representation.   You can changed the signal between signed and unsigned, and relocate the binary point.<P><P>Hardware notes: In hardware this block costs nothing.<P><P>Example:  Suppose the input is 6 bits wide, signed, with 2 fractional bits, and the output is forced to unsigned with 0 fractional bits.  Then an input of -2.0 (1110.00 in binary 2's complement) becomes an output of 56 (111000 in binary)."  block_version=10.1.1
  Reinterpret3 : xbsIndex_r4/Reinterpret  force_arith_type=on  arith_type=Unsigned  force_bin_pt=on  bin_pt=0  block_type=reinterpret
      settings: infoedit="Changes signal type without altering the binary representation.   You can changed the signal between signed and unsigned, and relocate the binary point.<P><P>Hardware notes: In hardware this block costs nothing.<P><P>Example:  Suppose the input is 6 bits wide, signed, with 2 fractional bits, and the output is forced to unsigned with 0 fractional bits.  Then an input of -2.0 (1110.00 in binary 2's complement) becomes an output of 56 (111000 in binary)."  block_version=10.1.1
  a0 : Subsystem  Tag=xps:bram  AncestorBlock=xps_library/Shared BRAM  mask{arith_type=Unsigned, addr_width=nsamples, data_width=32, data_bin_pt=0, init_vals=0, sample_rate=1}
      mask prompts: arith_type "Output Data Type"; addr_width "Address width"; data_width "Data Width"; data_bin_pt "Data Binary Point"; init_vals "Initial 32-bit values (simulation only)"; sample_rate "Sample rate"
      mask init:
      | shared_bram_mask;
      mask StyleString: popup(Unsigned|Signed  (2's comp)),edit,popup(8|16|32|64|128),edit,edit,edit
  a1 : Subsystem  Tag=xps:bram  AncestorBlock=xps_library/Shared BRAM  mask{arith_type=Unsigned, addr_width=nsamples, data_width=32, data_bin_pt=0, init_vals=0, sample_rate=1}
      mask prompts: arith_type "Output Data Type"; addr_width "Address width"; data_width "Data Width"; data_bin_pt "Data Binary Point"; init_vals "Initial 32-bit values (simulation only)"; sample_rate "Sample rate"
      mask init:
      | shared_bram_mask;
      mask StyleString: popup(Unsigned|Signed  (2's comp)),edit,popup(8|16|32|64|128),edit,edit,edit
  addr : xps_library/software register  Tag=xps:sw_reg  SystemSampleTime=-1  io_dir=To Processor  arith_type=Unsigned  bitwidth=32  bin_pt=0  sample_period=1  gw_name=v01_ssg_only_adcsnap_addr_user_data_in
  b0 : Subsystem  Tag=xps:bram  AncestorBlock=xps_library/Shared BRAM  mask{arith_type=Unsigned, addr_width=nsamples, data_width=32, data_bin_pt=0, init_vals=0, sample_rate=1}
      mask prompts: arith_type "Output Data Type"; addr_width "Address width"; data_width "Data Width"; data_bin_pt "Data Binary Point"; init_vals "Initial 32-bit values (simulation only)"; sample_rate "Sample rate"
      mask init:
      | shared_bram_mask;
      mask StyleString: popup(Unsigned|Signed  (2's comp)),edit,popup(8|16|32|64|128),edit,edit,edit
  b1 : Subsystem  Tag=xps:bram  AncestorBlock=xps_library/Shared BRAM  mask{arith_type=Unsigned, addr_width=nsamples, data_width=32, data_bin_pt=0, init_vals=0, sample_rate=1}
      mask prompts: arith_type "Output Data Type"; addr_width "Address width"; data_width "Data Width"; data_bin_pt "Data Binary Point"; init_vals "Initial 32-bit values (simulation only)"; sample_rate "Sample rate"
      mask init:
      | shared_bram_mask;
      mask StyleString: popup(Unsigned|Signed  (2's comp)),edit,popup(8|16|32|64|128),edit,edit,edit
  ctrl : xps_library/software register  Tag=xps:sw_reg  SystemSampleTime=-1  io_dir=From Processor  arith_type=Unsigned  bitwidth=32  bin_pt=0  sample_period=1  gw_name=v01_ssg_only_adcsnap_ctrl_user_data_out
  en1 : xbsIndex_r4/Slice  nbits=32  boolean_output=off  mode=Lower Bit Location + Width  bit1=0  base1=LSB of Input  bit0=32  base0=LSB of Input  dbl_ovrd=off  block_type=slice
      settings: infoedit="Extracts a given range of bits from each input sample and presents it at the output.  The output type is ordinarily unsigned with binary point at zero, but can be Boolean when the slice is one bit wide.<P><P>Hardware notes: In hardware this block costs nothing."  block_version=10.1.1
  en2 : xbsIndex_r4/Slice  nbits=32  boolean_output=off  mode=Lower Bit Location + Width  bit1=0  base1=LSB of Input  bit0=0  base0=LSB of Input  dbl_ovrd=off  block_type=slice
      settings: infoedit="Extracts a given range of bits from each input sample and presents it at the output.  The output type is ordinarily unsigned with binary point at zero, but can be Boolean when the slice is one bit wide.<P><P>Hardware notes: In hardware this block costs nothing."  block_version=10.1.1
  en3 : xbsIndex_r4/Slice  nbits=32  boolean_output=off  mode=Lower Bit Location + Width  bit1=0  base1=LSB of Input  bit0=32  base0=LSB of Input  dbl_ovrd=off  block_type=slice
      settings: infoedit="Extracts a given range of bits from each input sample and presents it at the output.  The output type is ordinarily unsigned with binary point at zero, but can be Boolean when the slice is one bit wide.<P><P>Hardware notes: In hardware this block costs nothing."  block_version=10.1.1
  en4 : xbsIndex_r4/Slice  nbits=32  boolean_output=off  mode=Lower Bit Location + Width  bit1=0  base1=LSB of Input  bit0=0  base0=LSB of Input  dbl_ovrd=off  block_type=slice
      settings: infoedit="Extracts a given range of bits from each input sample and presents it at the output.  The output type is ordinarily unsigned with binary point at zero, but can be Boolean when the slice is one bit wide.<P><P>Hardware notes: In hardware this block costs nothing."  block_version=10.1.1
  enable : xbsIndex_r4/Slice  nbits=1  boolean_output=on  mode=Lower Bit Location + Width  bit1=0  base1=LSB of Input  bit0=0  base0=LSB of Input  dbl_ovrd=off  block_type=slice
      settings: infoedit="Extracts a given range of bits from each input sample and presents it at the output.  The output type is ordinarily unsigned with binary point at zero, but can be Boolean when the slice is one bit wide.<P><P>Hardware notes: In hardware this block costs nothing."  block_version=10.1.1
  freeze_cntr : casper_library_misc/freeze_cntr  SystemSampleTime=-1  CounterBits=nsamples
  posedge : casper_library_misc/posedge  Tag=Rising Edge Detector  SystemSampleTime=-1
  trig1 : xbsIndex_r4/Slice  nbits=1  boolean_output=on  mode=Lower Bit Location + Width  bit1=0  base1=LSB of Input  bit0=1  base0=LSB of Input  dbl_ovrd=off  block_type=slice
      settings: infoedit="Extracts a given range of bits from each input sample and presents it at the output.  The output type is ordinarily unsigned with binary point at zero, but can be Boolean when the slice is one bit wide.<P><P>Hardware notes: In hardware this block costs nothing."  block_version=10.1.1
  valid : xbsIndex_r4/Slice  nbits=1  boolean_output=on  mode=Lower Bit Location + Width  bit1=0  base1=LSB of Input  bit0=2  base0=LSB of Input  dbl_ovrd=off  block_type=slice
      settings: infoedit="Extracts a given range of bits from each input sample and presents it at the output.  The output type is ordinarily unsigned with binary point at zero, but can be Boolean when the slice is one bit wide.<P><P>Hardware notes: In hardware this block costs nothing."  block_version=10.1.1
  wires:
  freeze_cntr/1 -> b1/1(addr), b0/1(addr), a1/1(addr), a0/1(addr), Register1/1
  Register/1 -> freeze_cntr/2
  Mux2/1 -> Logical1/1
  Inverter/1 -> Logical1/2
  Logical1/1 -> Register/2
  valid/1 -> Mux1/1
  trig1/1 -> Mux2/1
  Register1/1 -> addr/1
  Constant2/1 -> Mux1/3
  we/1 -> Mux1/2
  Mux1/1 -> freeze_cntr/1
  Constant1/1 -> Mux2/3
  Constant/1 -> Register/1
  posedge/1 -> Inverter/1, Register1/2, Register/3
  ctrl/1 -> trig1/1, valid/1, enable/1
  Constant13/1 -> ctrl/1
  freeze_cntr/2 -> b1/3(we), b0/3(we), a1/3(we), a0/3(we), Register1/3
  enable/1 -> posedge/1
  trig/1 -> Mux2/2
  Reinterpret3/1 -> en1/1, en2/1
  adcB/1 -> Reinterpret3/1
  en1/1 -> b0/2(data_in)
  en2/1 -> b1/2(data_in)
  Reinterpret1/1 -> en3/1, en4/1
  adcA/1 -> Reinterpret1/1
  en3/1 -> a0/2(data_in)
  en4/1 -> a1/2(data_in)

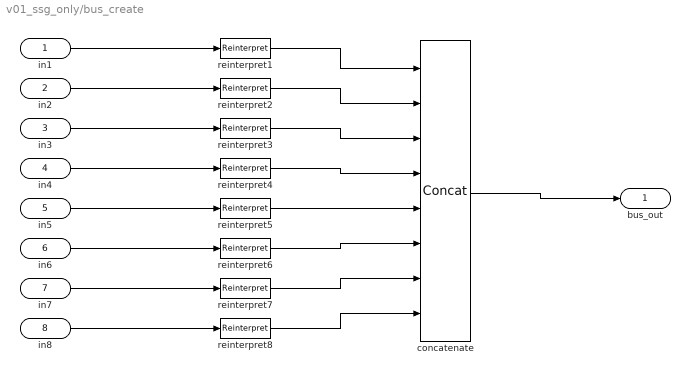
== system v01_ssg_only/bus_create ==
  in1 : Inport
  in2 : Inport  Port=2
  in3 : Inport  Port=3
  in4 : Inport  Port=4
  in5 : Inport  Port=5
  in6 : Inport  Port=6
  in7 : Inport  Port=7
  in8 : Inport  Port=8
  concatenate : xbsIndex_r4/Concat  num_inputs=8  dbl_ovrd=off  block_type=concat
  reinterpret{1..8} (8 alike) : xbsIndex_r4/Reinterpret  force_arith_type=on  arith_type=Unsigned  force_bin_pt=on  bin_pt=0  block_type=reinterpret
      reinterpret1 settings: infoedit="Changes signal type without altering the binary representation.   You can changed the signal between signed and unsigned, and relocate the binary point.<br><br>Hardware notes: In hardware this block costs nothing.<br><br>Example:  Suppose the input is 6 bits wide, signed, with 2 fractional bits, and the output is forced to unsigned with 0 fractional bits.  Then an input of -2.0 (1110.00 in binary 2's complement) becomes an output of 56 (111000 in binary)."
      reinterpret2 settings: infoedit="Changes signal type without altering the binary representation.   You can changed the signal between signed and unsigned, and relocate the binary point.<br><br>Hardware notes: In hardware this block costs nothing.<br><br>Example:  Suppose the input is 6 bits wide, signed, with 2 fractional bits, and the output is forced to unsigned with 0 fractional bits.  Then an input of -2.0 (1110.00 in binary 2's complement) becomes an output of 56 (111000 in binary)."
  bus_out : Outport
  wires:
  concatenate/1 -> bus_out/1
  in1/1 -> reinterpret1/1
  reinterpret1/1 -> concatenate/1
  in2/1 -> reinterpret2/1
  reinterpret2/1 -> concatenate/2
  in3/1 -> reinterpret3/1
  reinterpret3/1 -> concatenate/3
  in4/1 -> reinterpret4/1
  reinterpret4/1 -> concatenate/4
  in5/1 -> reinterpret5/1
  reinterpret5/1 -> concatenate/5
  in6/1 -> reinterpret6/1
  reinterpret6/1 -> concatenate/6
  in7/1 -> reinterpret7/1
  reinterpret7/1 -> concatenate/7
  in8/1 -> reinterpret8/1
  reinterpret8/1 -> concatenate/8

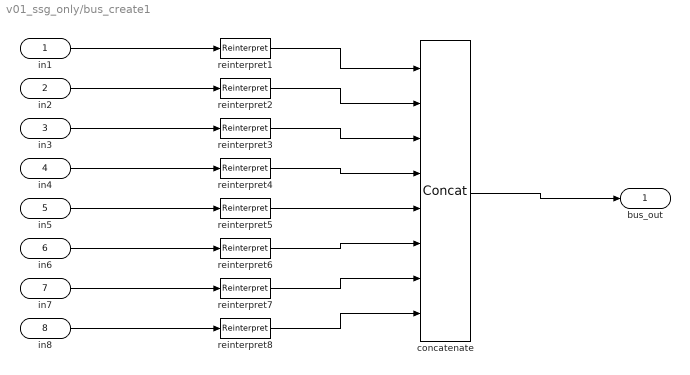
== system v01_ssg_only/bus_create1 ==
  in1 : Inport
  in2 : Inport  Port=2
  in3 : Inport  Port=3
  in4 : Inport  Port=4
  in5 : Inport  Port=5
  in6 : Inport  Port=6
  in7 : Inport  Port=7
  in8 : Inport  Port=8
  concatenate : xbsIndex_r4/Concat  num_inputs=8  dbl_ovrd=off  block_type=concat
  reinterpret{1..8} (8 alike) : xbsIndex_r4/Reinterpret  force_arith_type=on  arith_type=Unsigned  force_bin_pt=on  bin_pt=0  block_type=reinterpret
      reinterpret1 settings: infoedit="Changes signal type without altering the binary representation.   You can changed the signal between signed and unsigned, and relocate the binary point.<br><br>Hardware notes: In hardware this block costs nothing.<br><br>Example:  Suppose the input is 6 bits wide, signed, with 2 fractional bits, and the output is forced to unsigned with 0 fractional bits.  Then an input of -2.0 (1110.00 in binary 2's complement) becomes an output of 56 (111000 in binary)."
      reinterpret2 settings: infoedit="Changes signal type without altering the binary representation.   You can changed the signal between signed and unsigned, and relocate the binary point.<br><br>Hardware notes: In hardware this block costs nothing.<br><br>Example:  Suppose the input is 6 bits wide, signed, with 2 fractional bits, and the output is forced to unsigned with 0 fractional bits.  Then an input of -2.0 (1110.00 in binary 2's complement) becomes an output of 56 (111000 in binary)."
  bus_out : Outport
  wires:
  concatenate/1 -> bus_out/1
  in1/1 -> reinterpret1/1
  reinterpret1/1 -> concatenate/1
  in2/1 -> reinterpret2/1
  reinterpret2/1 -> concatenate/2
  in3/1 -> reinterpret3/1
  reinterpret3/1 -> concatenate/3
  in4/1 -> reinterpret4/1
  reinterpret4/1 -> concatenate/4
  in5/1 -> reinterpret5/1
  reinterpret5/1 -> concatenate/5
  in6/1 -> reinterpret6/1
  reinterpret6/1 -> concatenate/6
  in7/1 -> reinterpret7/1
  reinterpret7/1 -> concatenate/7
  in8/1 -> reinterpret8/1
  reinterpret8/1 -> concatenate/8
